simulink library "tp333079"  (Simulink 5.0)
values from neighbouring files (symbols this model uses):
  b = 1    [main_flock3.m]    (also in main_flock4.m; params_flocking_ros.m)
undefined symbols (not defined in the file or in its folder): AC, AlphaBnd, BetaBnd, CDda, CDde, CDdf, CDdr, CDM, CDmin, CGempty, CGgross, CL0, CLa, CLalphadot, Clbeta, Clda, CLde, CLdf, Cldr, CLM, CLmind, Clp, CLq, Clr, Cm0, Cma, Cmalphadot, Cmde, Cmdf, CmM, Cmq, Cnbeta, Cnda, Cndr, Cnp, Cnr, CP, CT, CYbeta, CYda, CYdr, CYp, CYr, Displacement, dmy, Engine, EulerIni, FuelFlow, FuelIni, J, Jempty, Jeng, Jgross, Jprop, MAC, MAP, MAPLim, MassIni, MaxPower, mempty ... (+26)
libraries: aerosimlib x325, simulink3 x42
(part 9 of 11)

== system tp333079/FlightGear-Compatible/Propulsion/Thruster/Propeller ==
  FG Fixed-Pitch Propeller : Subsystem  SimViewingDevice=off  mask(FG Fixed-pitch propeller model){Thr=Thruster}
      mask prompts: Thr "Thruster structure:"
      mask help: Fixed-pitch propeller model using look-up tables of thrust and power coefficients as functions of advance ratio.
      settings: Permissions=ReadWrite  RTWFcnNameOpts=Auto  RTWFileNameOpts=Auto
      mask Help:
      | The block provides a fixed-pitch propeller model based on look-up tables for thrust and power coefficients as function of the advance ratio.
      | <P><B>Inputs:</B>
      | <LI>Airspeed = the current aircraft airspeed</LI>
      | <LI>rho = the air density at current aircraft altitude</LI>
      | <LI>Omega = the propeller rotation speed</LI>
      | </P>
      | <P><B>Output:</B>
      | <LI>Fprop = the thrust force generated by the propeller (on body x-axis)</LI>
      | <LI>Mprop = the moment generated by the propeller (on body x-axis)</LI>
      | <LI>PropCoeff = the 3x1 vector of propeller coefficients [J CT CP]</LI>
      | </P>
      | <P><B>Parameters:</B>
      | <LI>Thruster structure = the thruster structure which is a part of the Matlab structure</LI>
      | </P>
  FG Variable-Pitch Propeller : Subsystem  SimViewingDevice=off  mask(FG Variable-pitch propeller model){Thr=Thr}
      mask prompts: Thr "Thruster structure:"
      mask help: Variable-pitch propeller model using look-up tables of thrust and power coefficients as functions of advance ratio and pitch angle.
      settings: Permissions=ReadWrite  RTWFcnNameOpts=Auto  RTWFileNameOpts=Auto
      mask Help:
      | The block provides a variable-pitch propeller model based on look-up tables for thrust and power coefficients as function of the advance ratio and blade pitch angle.
      | <P><B>Inputs:</B>
      | <LI>Airspeed = the current aircraft airspeed</LI>
      | <LI>rho = the air density at current aircraft altitude</LI>
      | <LI>Omega = the propeller rotation speed</LI>
      | <LI>Pitch = the prop blade pitch angle</LI>
      | </P>
      | <P><B>Output:</B>
      | <LI>Fprop = the thrust force generated by the propeller (on body x-axis)</LI>
      | <LI>Mprop = the moment generated by the propeller (on body x-axis)</LI>
      | <LI>PropCoeff = the 3x1 vector of propeller coefficients [J CT CP]</LI>
      | </P>
      | <P><B>Parameters:</B>
      | <LI>Thruster structure = the thruster structure which is a part of the aircraft structure.</LI>
      | </P>

== system tp333079/Equations of Motion/Body-Frame EOM/Kinematics (Quaternions)/Normalization/Vector norm ==
  Vec : Inport  Port=1  PortDimensions=-1  SampleTime=-1  DataType=auto
      settings: SignalType=auto
  Dot Product : simulink3/Math/Dot Product
  Math Function : Math  Operator=sqrt  OutputSignalType=auto
  Mag : Outport  Port=1
  wires:
  Math Function/1 -> Mag/1
  Dot Product/1 -> Math Function/1
  Vec/1 -> Dot Product/2, Dot Product/1

== system tp333079/FlightGear-Compatible/Complete Aircraft/CESSNA-172/Aerodynamics/Drag ==
  Control : Inport  Port=1  PortDimensions=[4 1]  SampleTime=-1  DataType=auto
      settings: SignalType=auto
  WindAxesVel : Inport  Port=2  PortDimensions=[3 1]  SampleTime=-1  DataType=auto
      settings: SignalType=auto
  GndEffect : Inport  Port=3  PortDimensions=1  SampleTime=-1  DataType=auto
      settings: SignalType=auto
  CD alpha : Subsystem  BlockChoice=Table  SimViewingDevice=off
      link override Table: Table=AC.Aerodynamics.Drag.Basic.CDwbh
      link override Value: Value=AC.Aerodynamics.Lift.Basic.kCLge
      link override Vector: Vector=AC.Aerodynamics.Lift.Basic.CLDf
      settings: AttributesFormatString=%<BlockChoice>  TemplateBlock=aerosimlib/FlightGear-Compatible/Aerodynamics/Coefficient  MemberBlocks=Table,Value,Vector  Permissions=ReadWrite  RTWFcnNameOpts=Auto  RTWFileNameOpts=Auto
  CD beta : Subsystem  BlockChoice=Value  SimViewingDevice=off
      link override Value: Value=AC.Aerodynamics.Drag.CDbeta
      settings: AttributesFormatString=%<BlockChoice>  TemplateBlock=aerosimlib/FlightGear-Compatible/Aerodynamics/Coefficient  MemberBlocks=Table,Value,Vector  Permissions=ReadWrite  RTWFcnNameOpts=Auto  RTWFileNameOpts=Auto
  CD elevator : Subsystem  BlockChoice=Value  SimViewingDevice=off
      link override Value: Value=AC.Aerodynamics.Drag.CDDe
      settings: AttributesFormatString=%<BlockChoice>  TemplateBlock=aerosimlib/FlightGear-Compatible/Aerodynamics/Coefficient  MemberBlocks=Table,Value,Vector  Permissions=ReadWrite  RTWFcnNameOpts=Auto  RTWFileNameOpts=Auto
  CD flap : Subsystem  BlockChoice=Vector  SimViewingDevice=off
      link override Value: Value=AC.Aerodynamics.Lift.Basic.kCLge
      link override Vector: Vector=AC.Aerodynamics.Drag.Basic.CDDf
      settings: AttributesFormatString=%<BlockChoice>  TemplateBlock=aerosimlib/FlightGear-Compatible/Aerodynamics/Coefficient  MemberBlocks=Table,Value,Vector  Permissions=ReadWrite  RTWFcnNameOpts=Auto  RTWFileNameOpts=Auto
  CDo : Constant  Value=AC.Aerodynamics.Drag.CDo.Data
  Demux : Demux  Outputs=4  BusSelectionMode=off
  Demux1 : Demux  Outputs=3  BusSelectionMode=off
  Product : Product  Inputs=2  Multiplication=Element-wise(.*)  SaturateOnIntegerOverflow=on
  Sum : Sum  Inputs=++  SaturateOnIntegerOverflow=on
  Sum1 : Sum  Inputs=++++  SaturateOnIntegerOverflow=on
  Terminator : Terminator
  Terminator1 : Terminator
  Terminator5 : Terminator
  kCD ground effect : Subsystem  BlockChoice=Vector  SimViewingDevice=off
      link override Value: Value=AC.Aerodynamics.Lift.Basic.kCLge
      link override Vector: Vector=AC.Aerodynamics.Drag.Basic.kCDge
      settings: AttributesFormatString=%<BlockChoice>  TemplateBlock=aerosimlib/FlightGear-Compatible/Aerodynamics/Coefficient  MemberBlocks=Table,Value,Vector  Permissions=ReadWrite  RTWFcnNameOpts=Auto  RTWFileNameOpts=Auto
  CD : Outport  Port=1
  wires:
  Demux/2 -> CD elevator/1(RowParam)
  WindAxesVel/1 -> Demux1/1
  Control/1 -> Demux/1
  Demux/1 -> CD alpha/2(ColParam), CD flap/1(RowParam)
  Demux/3 -> Terminator/1
  Demux/4 -> Terminator1/1
  Demux1/3 -> CD alpha/1(RowParam)
  CD alpha/1(Coeff) -> Sum/1
  CD flap/1(Coeff) -> Sum/2
  Sum/1 -> Product/1
  kCD ground effect/1(Coeff) -> Product/2
  Product/1 -> Sum1/1
  CDo/1 -> Sum1/2
  CD elevator/1(Coeff) -> Sum1/3
  CD beta/1(Coeff) -> Sum1/4
  Sum1/1 -> CD/1
  Demux1/1 -> Terminator5/1
  Demux1/2 -> CD beta/1(RowParam)
  GndEffect/1 -> kCD ground effect/1(RowParam)

== system tp333079/FlightGear-Compatible/Complete Aircraft/CESSNA-172/Aerodynamics/Lift ==
  Control : Inport  Port=1  PortDimensions=[4 1]  SampleTime=-1  DataType=auto
      settings: SignalType=auto
  WindAxesVel : Inport  Port=2  PortDimensions=[3 1]  SampleTime=-1  DataType=auto
      settings: SignalType=auto
  AlphaBetaDot : Inport  Port=3  PortDimensions=[2 1]  SampleTime=-1  DataType=auto
      settings: SignalType=auto
  AngularRates : Inport  Port=4  PortDimensions=[3 1]  SampleTime=-1  DataType=auto
      settings: SignalType=auto
  HystParam : Inport  Port=5  PortDimensions=1  SampleTime=-1  DataType=auto
      settings: SignalType=auto
  GndEffect : Inport  Port=6  PortDimensions=1  SampleTime=-1  DataType=auto
      settings: SignalType=auto
  2 : Gain  Gain=2  Multiplication=Element-wise(K.*u)  SaturateOnIntegerOverflow=on
  CL alpha : Subsystem  BlockChoice=Table  SimViewingDevice=off
      link override Table: Table=AC.Aerodynamics.Lift.Basic.CLwbh
      link override Value: Value=AC.Aerodynamics.Lift.Basic.kCLge
      link override Vector: Vector=AC.Aerodynamics.Lift.Basic.CLDf
      settings: AttributesFormatString=%<BlockChoice>  TemplateBlock=aerosimlib/FlightGear-Compatible/Aerodynamics/Coefficient  MemberBlocks=Table,Value,Vector  Permissions=ReadWrite  RTWFcnNameOpts=Auto  RTWFileNameOpts=Auto
  CL elevator : Subsystem  BlockChoice=Value  SimViewingDevice=off
      link override Value: Value=AC.Aerodynamics.Lift.CLDe
      settings: AttributesFormatString=%<BlockChoice>  TemplateBlock=aerosimlib/FlightGear-Compatible/Aerodynamics/Coefficient  MemberBlocks=Table,Value,Vector  Permissions=ReadWrite  RTWFcnNameOpts=Auto  RTWFileNameOpts=Auto
  CL flap : Subsystem  BlockChoice=Vector  SimViewingDevice=off
      link override Value: Value=AC.Aerodynamics.Lift.Basic.kCLge
      link override Vector: Vector=AC.Aerodynamics.Lift.Basic.CLDf
      settings: AttributesFormatString=%<BlockChoice>  TemplateBlock=aerosimlib/FlightGear-Compatible/Aerodynamics/Coefficient  MemberBlocks=Table,Value,Vector  Permissions=ReadWrite  RTWFcnNameOpts=Auto  RTWFileNameOpts=Auto
  CL*c/(2V) : Product  Inputs=**/  Multiplication=Element-wise(.*)  SaturateOnIntegerOverflow=on
  CLalphadot : Subsystem  BlockChoice=Value  SimViewingDevice=off
      link override Value: Value=AC.Aerodynamics.Lift.CLadot
      settings: AttributesFormatString=%<BlockChoice>  TemplateBlock=aerosimlib/FlightGear-Compatible/Aerodynamics/Coefficient  MemberBlocks=Table,Value,Vector  Permissions=ReadWrite  RTWFcnNameOpts=Auto  RTWFileNameOpts=Auto
  CLq : Subsystem  BlockChoice=Value  SimViewingDevice=off
      link override Value: Value=AC.Aerodynamics.Lift.CLq
      settings: AttributesFormatString=%<BlockChoice>  TemplateBlock=aerosimlib/FlightGear-Compatible/Aerodynamics/Coefficient  MemberBlocks=Table,Value,Vector  Permissions=ReadWrite  RTWFcnNameOpts=Auto  RTWFileNameOpts=Auto
  Demux : Demux  Outputs=4  BusSelectionMode=off
  Demux1 : Demux  Outputs=3  BusSelectionMode=off
  Demux2 : Demux  Outputs=2  BusSelectionMode=off
  Demux3 : Demux  Outputs=3  BusSelectionMode=off
  Product : Product  Inputs=2  Multiplication=Element-wise(.*)  SaturateOnIntegerOverflow=on
  Sum : Sum  Inputs=++  SaturateOnIntegerOverflow=on
  Sum1 : Sum  Inputs=+++  SaturateOnIntegerOverflow=on
  Sum2 : Sum  Inputs=++  SaturateOnIntegerOverflow=on
  Terminator{,1..4,6} (6 alike) : Terminator
  Wing chord : Constant  Value=AC.Metrics.WingChord
  kCL ground effect : Subsystem  BlockChoice=Vector  SimViewingDevice=off
      link override Value: Value=AC.Aerodynamics.Lift.Basic.kCLge
      link override Vector: Vector=AC.Aerodynamics.Lift.Basic.kCLge
      settings: AttributesFormatString=%<BlockChoice>  TemplateBlock=aerosimlib/FlightGear-Compatible/Aerodynamics/Coefficient  MemberBlocks=Table,Value,Vector  Permissions=ReadWrite  RTWFcnNameOpts=Auto  RTWFileNameOpts=Auto
  CL : Outport  Port=1
  wires:
  CL*c/(2V)/1 -> Sum1/3
  CLq/1(Coeff) -> Sum2/2
  CLalphadot/1(Coeff) -> Sum2/1
  Sum2/1 -> CL*c/(2V)/1
  Wing chord/1 -> CL*c/(2V)/2
  2/1 -> CL*c/(2V)/3
  GndEffect/1 -> kCL ground effect/1(RowParam)
  HystParam/1 -> CL alpha/2(ColParam)
  Demux1/2 -> Terminator6/1
  Demux1/1 -> 2/1
  Sum1/1 -> CL/1
  CL elevator/1(Coeff) -> Sum1/2
  Product/1 -> Sum1/1
  kCL ground effect/1(Coeff) -> Product/2
  Sum/1 -> Product/1
  CL flap/1(Coeff) -> Sum/2
  CL alpha/1(Coeff) -> Sum/1
  Demux3/3 -> Terminator4/1
  Demux3/1 -> Terminator3/1
  Demux2/2 -> Terminator2/1
  Demux3/2 -> CLq/1(RowParam)
  Demux2/1 -> CLalphadot/1(RowParam)
  Demux1/3 -> CL alpha/1(RowParam)
  Demux/4 -> Terminator1/1
  Demux/3 -> Terminator/1
  Demux/2 -> CL elevator/1(RowParam)
  Demux/1 -> CL flap/1(RowParam)
  AngularRates/1 -> Demux3/1
  AlphaBetaDot/1 -> Demux2/1
  Control/1 -> Demux/1
  WindAxesVel/1 -> Demux1/1

== system tp333079/FlightGear-Compatible/Complete Aircraft/CESSNA-172/Aerodynamics/Pitch ==
  Control : Inport  Port=1  PortDimensions=[4 1]  SampleTime=-1  DataType=auto
      settings: SignalType=auto
  WindAxesVel : Inport  Port=2  PortDimensions=[3 1]  SampleTime=-1  DataType=auto
      settings: SignalType=auto
  AlphaBetaDot : Inport  Port=3  PortDimensions=[2 1]  SampleTime=-1  DataType=auto
      settings: SignalType=auto
  AngularRates : Inport  Port=4  PortDimensions=[3 1]  SampleTime=-1  DataType=auto
      settings: SignalType=auto
  2 : Gain  Gain=2  Multiplication=Element-wise(K.*u)  SaturateOnIntegerOverflow=on
  Cm alpha : Subsystem  BlockChoice=Value  SimViewingDevice=off
      link override Table: Table=AC.Aerodynamics.Lift.Basic.CLwbh
      link override Value: Value=AC.Aerodynamics.Pitch.Cmalpha
      link override Vector: Vector=AC.Aerodynamics.Lift.Basic.CLDf
      settings: AttributesFormatString=%<BlockChoice>  TemplateBlock=aerosimlib/FlightGear-Compatible/Aerodynamics/Coefficient  MemberBlocks=Table,Value,Vector  Permissions=ReadWrite  RTWFcnNameOpts=Auto  RTWFileNameOpts=Auto
  Cm elevator : Subsystem  BlockChoice=Value  SimViewingDevice=off
      link override Value: Value=AC.Aerodynamics.Pitch.Cmde
      settings: AttributesFormatString=%<BlockChoice>  TemplateBlock=aerosimlib/FlightGear-Compatible/Aerodynamics/Coefficient  MemberBlocks=Table,Value,Vector  Permissions=ReadWrite  RTWFcnNameOpts=Auto  RTWFileNameOpts=Auto
  Cm flap : Subsystem  BlockChoice=Vector  SimViewingDevice=off
      link override Value: Value=AC.Aerodynamics.Lift.Basic.kCLge
      link override Vector: Vector=AC.Aerodynamics.Pitch.Cmdf
      settings: AttributesFormatString=%<BlockChoice>  TemplateBlock=aerosimlib/FlightGear-Compatible/Aerodynamics/Coefficient  MemberBlocks=Table,Value,Vector  Permissions=ReadWrite  RTWFcnNameOpts=Auto  RTWFileNameOpts=Auto
  Cm*c/(2V) : Product  Inputs=**/  Multiplication=Element-wise(.*)  SaturateOnIntegerOverflow=on
  Cmalphadot : Subsystem  BlockChoice=Value  SimViewingDevice=off
      link override Value: Value=AC.Aerodynamics.Pitch.Cmadot
      settings: AttributesFormatString=%<BlockChoice>  TemplateBlock=aerosimlib/FlightGear-Compatible/Aerodynamics/Coefficient  MemberBlocks=Table,Value,Vector  Permissions=ReadWrite  RTWFcnNameOpts=Auto  RTWFileNameOpts=Auto
  Cmo : Constant  Value=AC.Aerodynamics.Pitch.Cmo.Data
  Cmq : Subsystem  BlockChoice=Value  SimViewingDevice=off
      link override Value: Value=AC.Aerodynamics.Pitch.Cmq
      settings: AttributesFormatString=%<BlockChoice>  TemplateBlock=aerosimlib/FlightGear-Compatible/Aerodynamics/Coefficient  MemberBlocks=Table,Value,Vector  Permissions=ReadWrite  RTWFcnNameOpts=Auto  RTWFileNameOpts=Auto
  Demux : Demux  Outputs=4  BusSelectionMode=off
  Demux1 : Demux  Outputs=3  BusSelectionMode=off
  Demux2 : Demux  Outputs=2  BusSelectionMode=off
  Demux3 : Demux  Outputs=3  BusSelectionMode=off
  Sum1 : Sum  Inputs=+++++  SaturateOnIntegerOverflow=on
  Sum2 : Sum  Inputs=++  SaturateOnIntegerOverflow=on
  Terminator{,1..4,6} (6 alike) : Terminator
  Wing chord : Constant  Value=AC.Metrics.WingChord
  Cm : Outport  Port=1
  wires:
  Cm*c/(2V)/1 -> Sum1/5
  Cm elevator/1(Coeff) -> Sum1/4
  Cmo/1 -> Sum1/3
  Cm flap/1(Coeff) -> Sum1/2
  Cm alpha/1(Coeff) -> Sum1/1
  Demux3/2 -> Cmq/1(RowParam)
  Demux2/1 -> Cmalphadot/1(RowParam)
  Demux1/3 -> Cm alpha/1(RowParam)
  Demux1/1 -> 2/1
  Demux/2 -> Cm elevator/1(RowParam)
  Demux/1 -> Cm flap/1(RowParam)
  WindAxesVel/1 -> Demux1/1
  Control/1 -> Demux/1
  AlphaBetaDot/1 -> Demux2/1
  AngularRates/1 -> Demux3/1
  Demux/3 -> Terminator/1
  Demux/4 -> Terminator1/1
  Demux2/2 -> Terminator2/1
  Demux3/1 -> Terminator3/1
  Demux3/3 -> Terminator4/1
  Sum1/1 -> Cm/1
  Demux1/2 -> Terminator6/1
  2/1 -> Cm*c/(2V)/3
  Wing chord/1 -> Cm*c/(2V)/2
  Sum2/1 -> Cm*c/(2V)/1
  Cmalphadot/1(Coeff) -> Sum2/1
  Cmq/1(Coeff) -> Sum2/2

== system tp333079/FlightGear-Compatible/Complete Aircraft/CESSNA-172/Aerodynamics/Roll ==
  Control : Inport  Port=1  PortDimensions=[4 1]  SampleTime=-1  DataType=auto
      settings: SignalType=auto
  WindAxesVel : Inport  Port=2  PortDimensions=[3 1]  SampleTime=-1  DataType=auto
      settings: SignalType=auto
  AngularRates : Inport  Port=3  PortDimensions=[3 1]  SampleTime=-1  DataType=auto
      settings: SignalType=auto
  2 : Gain  Gain=2  Multiplication=Element-wise(K.*u)  SaturateOnIntegerOverflow=on
  Cl aileron : Subsystem  BlockChoice=Value  SimViewingDevice=off
      link override Value: Value=AC.Aerodynamics.Roll.ClDa
      settings: AttributesFormatString=%<BlockChoice>  TemplateBlock=aerosimlib/FlightGear-Compatible/Aerodynamics/Coefficient  MemberBlocks=Table,Value,Vector  Permissions=ReadWrite  RTWFcnNameOpts=Auto  RTWFileNameOpts=Auto
  Cl beta : Subsystem  BlockChoice=Vector  SimViewingDevice=off
      link override Value: Value=AC.Aerodynamics.Lift.Basic.kCLge
      link override Vector: Vector=AC.Aerodynamics.Roll.Clb
      settings: AttributesFormatString=%<BlockChoice>  TemplateBlock=aerosimlib/FlightGear-Compatible/Aerodynamics/Coefficient  MemberBlocks=Table,Value,Vector  Permissions=ReadWrite  RTWFcnNameOpts=Auto  RTWFileNameOpts=Auto
  Cl rudder : Subsystem  BlockChoice=Value  SimViewingDevice=off
      link override Value: Value=AC.Aerodynamics.Roll.Cldr
      settings: AttributesFormatString=%<BlockChoice>  TemplateBlock=aerosimlib/FlightGear-Compatible/Aerodynamics/Coefficient  MemberBlocks=Table,Value,Vector  Permissions=ReadWrite  RTWFcnNameOpts=Auto  RTWFileNameOpts=Auto
  Cl*b/(2V) : Product  Inputs=**/  Multiplication=Element-wise(.*)  SaturateOnIntegerOverflow=on
  Clp : Subsystem  BlockChoice=Value  SimViewingDevice=off
      link override Value: Value=AC.Aerodynamics.Roll.Clp
      settings: AttributesFormatString=%<BlockChoice>  TemplateBlock=aerosimlib/FlightGear-Compatible/Aerodynamics/Coefficient  MemberBlocks=Table,Value,Vector  Permissions=ReadWrite  RTWFcnNameOpts=Auto  RTWFileNameOpts=Auto
  Clr : Subsystem  BlockChoice=Table  SimViewingDevice=off
      link override Table: Table=AC.Aerodynamics.Roll.Clr
      link override Value: Value=AC.Aerodynamics.Side.CYdr
      link override Vector: Vector=AC.Aerodynamics.Roll.Clr
      settings: AttributesFormatString=%<BlockChoice>  TemplateBlock=aerosimlib/FlightGear-Compatible/Aerodynamics/Coefficient  MemberBlocks=Table,Value,Vector  Permissions=ReadWrite  RTWFcnNameOpts=Auto  RTWFileNameOpts=Auto
  Clr*r : Product  Inputs=2  Multiplication=Element-wise(.*)  SaturateOnIntegerOverflow=on
  Demux : Demux  Outputs=4  BusSelectionMode=off
  Demux1 : Demux  Outputs=3  BusSelectionMode=off
  Demux3 : Demux  Outputs=3  BusSelectionMode=off
  Sum : Sum  Inputs=++  SaturateOnIntegerOverflow=on
  Sum1 : Sum  Inputs=++++  SaturateOnIntegerOverflow=on
  Terminator3 : Terminator
  Terminator4 : Terminator
  Wing span : Constant  Value=AC.Metrics.WingSpan
  Cl : Outport  Port=1
  wires:
  Sum1/1 -> Cl/1
  AngularRates/1 -> Demux3/1
  Control/1 -> Demux/1
  WindAxesVel/1 -> Demux1/1
  Clp/1(Coeff) -> Sum/1
  Wing span/1 -> Cl*b/(2V)/2
  2/1 -> Cl*b/(2V)/3
  Sum/1 -> Cl*b/(2V)/1
  Demux1/1 -> 2/1
  Demux1/2 -> Cl beta/1(RowParam)
  Demux/3 -> Cl aileron/1(RowParam)
  Demux/4 -> Cl rudder/1(RowParam)
  Demux3/1 -> Clp/1(RowParam)
  Demux3/2 -> Terminator4/1
  Demux1/3 -> Clr/1(RowParam)
  Demux/1 -> Clr/2(ColParam)
  Demux/2 -> Terminator3/1
  Cl beta/1(Coeff) -> Sum1/1
  Cl aileron/1(Coeff) -> Sum1/2
  Cl rudder/1(Coeff) -> Sum1/3
  Cl*b/(2V)/1 -> Sum1/4
  Clr*r/1 -> Sum/2
  Clr/1(Coeff) -> Clr*r/1
  Demux3/3 -> Clr*r/2

== system tp333079/FlightGear-Compatible/Complete Aircraft/CESSNA-172/Aerodynamics/Side ==
  Control : Inport  Port=1  PortDimensions=[4 1]  SampleTime=-1  DataType=auto
      settings: SignalType=auto
  WindAxesVel : Inport  Port=2  PortDimensions=[3 1]  SampleTime=-1  DataType=auto
      settings: SignalType=auto
  AngularRates : Inport  Port=3  PortDimensions=[3 1]  SampleTime=-1  DataType=auto
      settings: SignalType=auto
  2 : Gain  Gain=2  Multiplication=Element-wise(K.*u)  SaturateOnIntegerOverflow=on
  CY aileron : Subsystem  BlockChoice=Value  SimViewingDevice=off
      link override Value: Value=AC.Aerodynamics.Side.CYda
      settings: AttributesFormatString=%<BlockChoice>  TemplateBlock=aerosimlib/FlightGear-Compatible/Aerodynamics/Coefficient  MemberBlocks=Table,Value,Vector  Permissions=ReadWrite  RTWFcnNameOpts=Auto  RTWFileNameOpts=Auto
  CY beta : Subsystem  BlockChoice=Table  SimViewingDevice=off
      link override Table: Table=AC.Aerodynamics.Side.CYb
      link override Value: Value=AC.Aerodynamics.Lift.Basic.kCLge
      link override Vector: Vector=AC.Aerodynamics.Side.CYb
      settings: AttributesFormatString=%<BlockChoice>  TemplateBlock=aerosimlib/FlightGear-Compatible/Aerodynamics/Coefficient  MemberBlocks=Table,Value,Vector  Permissions=ReadWrite  RTWFcnNameOpts=Auto  RTWFileNameOpts=Auto
  CY rudder : Subsystem  BlockChoice=Value  SimViewingDevice=off
      link override Value: Value=AC.Aerodynamics.Side.CYdr
      settings: AttributesFormatString=%<BlockChoice>  TemplateBlock=aerosimlib/FlightGear-Compatible/Aerodynamics/Coefficient  MemberBlocks=Table,Value,Vector  Permissions=ReadWrite  RTWFcnNameOpts=Auto  RTWFileNameOpts=Auto
  CY*b/(2V) : Product  Inputs=**/  Multiplication=Element-wise(.*)  SaturateOnIntegerOverflow=on
  CYp : Subsystem  BlockChoice=Table  SimViewingDevice=off
      link override Table: Table=AC.Aerodynamics.Side.CYp
      link override Value: Value=AC.Aerodynamics.Side.CYp
      settings: AttributesFormatString=%<BlockChoice>  TemplateBlock=aerosimlib/FlightGear-Compatible/Aerodynamics/Coefficient  MemberBlocks=Table,Value,Vector  Permissions=ReadWrite  RTWFcnNameOpts=Auto  RTWFileNameOpts=Auto
  CYr : Subsystem  BlockChoice=Table  SimViewingDevice=off
      link override Table: Table=AC.Aerodynamics.Side.CYr
      link override Value: Value=AC.Aerodynamics.Side.CYr
      settings: AttributesFormatString=%<BlockChoice>  TemplateBlock=aerosimlib/FlightGear-Compatible/Aerodynamics/Coefficient  MemberBlocks=Table,Value,Vector  Permissions=ReadWrite  RTWFcnNameOpts=Auto  RTWFileNameOpts=Auto
  Demux : Demux  Outputs=4  BusSelectionMode=off
  Demux1 : Demux  Outputs=3  BusSelectionMode=off
  Demux3 : Demux  Outputs=3  BusSelectionMode=off
  Product : Product  Inputs=2  Multiplication=Element-wise(.*)  SaturateOnIntegerOverflow=on
  Product1 : Product  Inputs=2  Multiplication=Element-wise(.*)  SaturateOnIntegerOverflow=on
  Sum : Sum  Inputs=++  SaturateOnIntegerOverflow=on
  Sum1 : Sum  Inputs=++++  SaturateOnIntegerOverflow=on
  Terminator3 : Terminator
  Terminator4 : Terminator
  Wing span : Constant  Value=AC.Metrics.WingSpan
  CY : Outport  Port=1
  wires:
  CY*b/(2V)/1 -> Sum1/4
  CY rudder/1(Coeff) -> Sum1/3
  CY aileron/1(Coeff) -> Sum1/2
  CY beta/1(Coeff) -> Sum1/1
  Demux/2 -> Terminator3/1
  Demux/1 -> CY beta/2(ColParam), CYp/2(ColParam), CYr/2(ColParam)
  Demux1/3 -> CYp/1(RowParam), CYr/1(RowParam)
  Demux3/2 -> Terminator4/1
  Demux/4 -> CY rudder/1(RowParam)
  Demux/3 -> CY aileron/1(RowParam)
  Demux1/2 -> CY beta/1(RowParam)
  Demux1/1 -> 2/1
  Sum/1 -> CY*b/(2V)/1
  2/1 -> CY*b/(2V)/3
  Wing span/1 -> CY*b/(2V)/2
  WindAxesVel/1 -> Demux1/1
  Control/1 -> Demux/1
  AngularRates/1 -> Demux3/1
  Sum1/1 -> CY/1
  Product/1 -> Sum/1
  Product1/1 -> Sum/2
  CYp/1(Coeff) -> Product/1
  CYr/1(Coeff) -> Product1/1
  Demux3/1 -> Product/2
  Demux3/3 -> Product1/2

== system tp333079/FlightGear-Compatible/Complete Aircraft/CESSNA-172/Aerodynamics/Yaw ==
  Control : Inport  Port=1  PortDimensions=[4 1]  SampleTime=-1  DataType=auto
      settings: SignalType=auto
  WindAxesVel : Inport  Port=2  PortDimensions=[3 1]  SampleTime=-1  DataType=auto
      settings: SignalType=auto
  AngularRates : Inport  Port=3  PortDimensions=[3 1]  SampleTime=-1  DataType=auto
      settings: SignalType=auto
  2 : Gain  Gain=2  Multiplication=Element-wise(K.*u)  SaturateOnIntegerOverflow=on
  Cn aileron : Subsystem  BlockChoice=Value  SimViewingDevice=off
      link override Value: Value=AC.Aerodynamics.Yaw.Cnda
      settings: AttributesFormatString=%<BlockChoice>  TemplateBlock=aerosimlib/FlightGear-Compatible/Aerodynamics/Coefficient  MemberBlocks=Table,Value,Vector  Permissions=ReadWrite  RTWFcnNameOpts=Auto  RTWFileNameOpts=Auto
  Cn beta : Subsystem  BlockChoice=Vector  SimViewingDevice=off
      link override Value: Value=AC.Aerodynamics.Lift.Basic.kCLge
      link override Vector: Vector=AC.Aerodynamics.Yaw.Cnb
      settings: AttributesFormatString=%<BlockChoice>  TemplateBlock=aerosimlib/FlightGear-Compatible/Aerodynamics/Coefficient  MemberBlocks=Table,Value,Vector  Permissions=ReadWrite  RTWFcnNameOpts=Auto  RTWFileNameOpts=Auto
  Cn rudder : Subsystem  BlockChoice=Value  SimViewingDevice=off
      link override Value: Value=AC.Aerodynamics.Yaw.Cndr
      settings: AttributesFormatString=%<BlockChoice>  TemplateBlock=aerosimlib/FlightGear-Compatible/Aerodynamics/Coefficient  MemberBlocks=Table,Value,Vector  Permissions=ReadWrite  RTWFcnNameOpts=Auto  RTWFileNameOpts=Auto
  Cn*b/(2V) : Product  Inputs=**/  Multiplication=Element-wise(.*)  SaturateOnIntegerOverflow=on
  Cnp : Subsystem  BlockChoice=Value  SimViewingDevice=off
      link override Value: Value=AC.Aerodynamics.Yaw.Cnp
      settings: AttributesFormatString=%<BlockChoice>  TemplateBlock=aerosimlib/FlightGear-Compatible/Aerodynamics/Coefficient  MemberBlocks=Table,Value,Vector  Permissions=ReadWrite  RTWFcnNameOpts=Auto  RTWFileNameOpts=Auto
  Cnr : Subsystem  BlockChoice=Value  SimViewingDevice=off
      link override Value: Value=AC.Aerodynamics.Yaw.Cnr
      link override Vector: Vector=AC.Aerodynamics.Roll.Clr
      settings: AttributesFormatString=%<BlockChoice>  TemplateBlock=aerosimlib/FlightGear-Compatible/Aerodynamics/Coefficient  MemberBlocks=Table,Value,Vector  Permissions=ReadWrite  RTWFcnNameOpts=Auto  RTWFileNameOpts=Auto
  Demux : Demux  Outputs=4  BusSelectionMode=off
  Demux1 : Demux  Outputs=3  BusSelectionMode=off
  Demux3 : Demux  Outputs=3  BusSelectionMode=off
  Sum : Sum  Inputs=++  SaturateOnIntegerOverflow=on
  Sum1 : Sum  Inputs=++++  SaturateOnIntegerOverflow=on
  Terminator{1..4} (4 alike) : Terminator
  Wing span : Constant  Value=AC.Metrics.WingSpan
  Cn : Outport  Port=1
  wires:
  Cn*b/(2V)/1 -> Sum1/4
  Cn rudder/1(Coeff) -> Sum1/3
  Cn aileron/1(Coeff) -> Sum1/2
  Cn beta/1(Coeff) -> Sum1/1
  Demux/2 -> Terminator3/1
  Demux/1 -> Terminator2/1
  Demux1/3 -> Terminator1/1
  Demux3/2 -> Terminator4/1
  Demux3/3 -> Cnr/1(RowParam)
  Demux3/1 -> Cnp/1(RowParam)
  Demux/4 -> Cn rudder/1(RowParam)
  Demux/3 -> Cn aileron/1(RowParam)
  Demux1/2 -> Cn beta/1(RowParam)
  Demux1/1 -> 2/1
  Sum/1 -> Cn*b/(2V)/1
  2/1 -> Cn*b/(2V)/3
  Wing span/1 -> Cn*b/(2V)/2
  Cnr/1(Coeff) -> Sum/2
  Cnp/1(Coeff) -> Sum/1
  WindAxesVel/1 -> Demux1/1
  Control/1 -> Demux/1
  AngularRates/1 -> Demux3/1
  Sum1/1 -> Cn/1

== system tp333079/FlightGear-Compatible/Complete Aircraft/CESSNA-182/Aerodynamics/Drag ==
  Control : Inport  Port=1  PortDimensions=[4 1]  SampleTime=-1  DataType=auto
      settings: SignalType=auto
  WindAxesVel : Inport  Port=2  PortDimensions=[3 1]  SampleTime=-1  DataType=auto
      settings: SignalType=auto
  CD alpha : Subsystem  BlockChoice=Vector  SimViewingDevice=off
      link override Table: Table=AC.Aerodynamics.Drag.Basic.CDwbh
      link override Value: Value=AC.Aerodynamics.Lift.Basic.kCLge
      link override Vector: Vector=AC.Aerodynamics.Drag.CDalpha
      settings: AttributesFormatString=%<BlockChoice>  TemplateBlock=aerosimlib/FlightGear-Compatible/Aerodynamics/Coefficient  MemberBlocks=Table,Value,Vector  Permissions=ReadWrite  RTWFcnNameOpts=Auto  RTWFileNameOpts=Auto
  CD beta : Subsystem  BlockChoice=Value  SimViewingDevice=off
      link override Value: Value=AC.Aerodynamics.Drag.CDbeta
      settings: AttributesFormatString=%<BlockChoice>  TemplateBlock=aerosimlib/FlightGear-Compatible/Aerodynamics/Coefficient  MemberBlocks=Table,Value,Vector  Permissions=ReadWrite  RTWFcnNameOpts=Auto  RTWFileNameOpts=Auto
  CD elevator : Subsystem  BlockChoice=Value  SimViewingDevice=off
      link override Value: Value=AC.Aerodynamics.Drag.CDDe
      settings: AttributesFormatString=%<BlockChoice>  TemplateBlock=aerosimlib/FlightGear-Compatible/Aerodynamics/Coefficient  MemberBlocks=Table,Value,Vector  Permissions=ReadWrite  RTWFcnNameOpts=Auto  RTWFileNameOpts=Auto
  CD flap : Subsystem  BlockChoice=Table  SimViewingDevice=off
      link override Table: Table=AC.Aerodynamics.Drag.CDDf
      link override Value: Value=AC.Aerodynamics.Lift.Basic.kCLge
      link override Vector: Vector=AC.Aerodynamics.Drag.Basic.CDDf
      settings: AttributesFormatString=%<BlockChoice>  TemplateBlock=aerosimlib/FlightGear-Compatible/Aerodynamics/Coefficient  MemberBlocks=Table,Value,Vector  Permissions=ReadWrite  RTWFcnNameOpts=Auto  RTWFileNameOpts=Auto
  CDo : Constant  Value=AC.Aerodynamics.Drag.CDo.Data
  Demux : Demux  Outputs=4  BusSelectionMode=off
  Demux1 : Demux  Outputs=3  BusSelectionMode=off
  Sum : Sum  Inputs=++  SaturateOnIntegerOverflow=on
  Sum1 : Sum  Inputs=++++  SaturateOnIntegerOverflow=on
  Terminator : Terminator
  Terminator1 : Terminator
  Terminator5 : Terminator
  CD : Outport  Port=1
  wires:
  Demux/1 -> CD flap/2(ColParam)
  Demux/2 -> CD elevator/1(RowParam)
  WindAxesVel/1 -> Demux1/1
  Control/1 -> Demux/1
  Demux/3 -> Terminator/1
  Demux/4 -> Terminator1/1
  Demux1/3 -> CD flap/1(RowParam), CD alpha/1(RowParam)
  CD alpha/1(Coeff) -> Sum/1
  CD flap/1(Coeff) -> Sum/2
  Sum/1 -> Sum1/1
  CDo/1 -> Sum1/2
  CD elevator/1(Coeff) -> Sum1/3
  CD beta/1(Coeff) -> Sum1/4
  Sum1/1 -> CD/1
  Demux1/1 -> Terminator5/1
  Demux1/2 -> CD beta/1(RowParam)

== system tp333079/FlightGear-Compatible/Complete Aircraft/CESSNA-182/Aerodynamics/Lift ==
  Control : Inport  Port=1  PortDimensions=[4 1]  SampleTime=-1  DataType=auto
      settings: SignalType=auto
  WindAxesVel : Inport  Port=2  PortDimensions=[3 1]  SampleTime=-1  DataType=auto
      settings: SignalType=auto
  AlphaBetaDot : Inport  Port=3  PortDimensions=[2 1]  SampleTime=-1  DataType=auto
      settings: SignalType=auto
  AngularRates : Inport  Port=4  PortDimensions=[3 1]  SampleTime=-1  DataType=auto
      settings: SignalType=auto
  GndEffect : Inport  Port=5  PortDimensions=1  SampleTime=-1  DataType=auto
      settings: SignalType=auto
  2 : Gain  Gain=2  Multiplication=Element-wise(K.*u)  SaturateOnIntegerOverflow=on
  CL alpha : Subsystem  BlockChoice=Vector  SimViewingDevice=off
      link override Table: Table=AC.Aerodynamics.Lift.Basic.CLalpha
      link override Value: Value=AC.Aerodynamics.Lift.Basic.kCLge
      link override Vector: Vector=AC.Aerodynamics.Lift.Basic.CLalpha
      settings: AttributesFormatString=%<BlockChoice>  TemplateBlock=aerosimlib/FlightGear-Compatible/Aerodynamics/Coefficient  MemberBlocks=Table,Value,Vector  Permissions=ReadWrite  RTWFcnNameOpts=Auto  RTWFileNameOpts=Auto
  CL elevator : Subsystem  BlockChoice=Value  SimViewingDevice=off
      link override Value: Value=AC.Aerodynamics.Lift.CLDe
      settings: AttributesFormatString=%<BlockChoice>  TemplateBlock=aerosimlib/FlightGear-Compatible/Aerodynamics/Coefficient  MemberBlocks=Table,Value,Vector  Permissions=ReadWrite  RTWFcnNameOpts=Auto  RTWFileNameOpts=Auto
  CL flap : Subsystem  BlockChoice=Vector  SimViewingDevice=off
      link override Value: Value=AC.Aerodynamics.Lift.Basic.kCLge
      link override Vector: Vector=AC.Aerodynamics.Lift.Basic.CLDf
      settings: AttributesFormatString=%<BlockChoice>  TemplateBlock=aerosimlib/FlightGear-Compatible/Aerodynamics/Coefficient  MemberBlocks=Table,Value,Vector  Permissions=ReadWrite  RTWFcnNameOpts=Auto  RTWFileNameOpts=Auto
  CL*c/(2V) : Product  Inputs=**/  Multiplication=Element-wise(.*)  SaturateOnIntegerOverflow=on
  CLalphadot : Subsystem  BlockChoice=Value  SimViewingDevice=off
      link override Value: Value=AC.Aerodynamics.Lift.CLadot
      settings: AttributesFormatString=%<BlockChoice>  TemplateBlock=aerosimlib/FlightGear-Compatible/Aerodynamics/Coefficient  MemberBlocks=Table,Value,Vector  Permissions=ReadWrite  RTWFcnNameOpts=Auto  RTWFileNameOpts=Auto
  CLo : Constant  Value=AC.Aerodynamics.Lift.Basic.CLo.Data
  CLq : Subsystem  BlockChoice=Value  SimViewingDevice=off
      link override Value: Value=AC.Aerodynamics.Lift.CLq
      settings: AttributesFormatString=%<BlockChoice>  TemplateBlock=aerosimlib/FlightGear-Compatible/Aerodynamics/Coefficient  MemberBlocks=Table,Value,Vector  Permissions=ReadWrite  RTWFcnNameOpts=Auto  RTWFileNameOpts=Auto
  Demux : Demux  Outputs=4  BusSelectionMode=off
  Demux1 : Demux  Outputs=3  BusSelectionMode=off
  Demux2 : Demux  Outputs=2  BusSelectionMode=off
  Demux3 : Demux  Outputs=3  BusSelectionMode=off
  Product : Product  Inputs=2  Multiplication=Element-wise(.*)  SaturateOnIntegerOverflow=on
  Sum : Sum  Inputs=+++  SaturateOnIntegerOverflow=on
  Sum1 : Sum  Inputs=+++  SaturateOnIntegerOverflow=on
  Sum2 : Sum  Inputs=++  SaturateOnIntegerOverflow=on
  Terminator{,1..4,6} (6 alike) : Terminator
  Wing chord : Constant  Value=AC.Metrics.WingChord
  kCL ground effect : Subsystem  BlockChoice=Vector  SimViewingDevice=off
      link override Value: Value=AC.Aerodynamics.Lift.Basic.kCLge
      link override Vector: Vector=AC.Aerodynamics.Lift.Basic.kCLge
      settings: AttributesFormatString=%<BlockChoice>  TemplateBlock=aerosimlib/FlightGear-Compatible/Aerodynamics/Coefficient  MemberBlocks=Table,Value,Vector  Permissions=ReadWrite  RTWFcnNameOpts=Auto  RTWFileNameOpts=Auto
  CL : Outport  Port=1
  wires:
  CLo/1 -> Sum/3
  CL*c/(2V)/1 -> Sum1/3
  CLq/1(Coeff) -> Sum2/2
  CLalphadot/1(Coeff) -> Sum2/1
  Sum2/1 -> CL*c/(2V)/1
  Wing chord/1 -> CL*c/(2V)/2
  2/1 -> CL*c/(2V)/3
  GndEffect/1 -> kCL ground effect/1(RowParam)
  Demux1/2 -> Terminator6/1
  Demux1/1 -> 2/1
  Sum1/1 -> CL/1
  CL elevator/1(Coeff) -> Sum1/2
  Product/1 -> Sum1/1
  kCL ground effect/1(Coeff) -> Product/2
  Sum/1 -> Product/1
  CL flap/1(Coeff) -> Sum/2
  CL alpha/1(Coeff) -> Sum/1
  Demux3/3 -> Terminator4/1
  Demux3/1 -> Terminator3/1
  Demux2/2 -> Terminator2/1
  Demux3/2 -> CLq/1(RowParam)
  Demux2/1 -> CLalphadot/1(RowParam)
  Demux1/3 -> CL alpha/1(RowParam)
  Demux/4 -> Terminator1/1
  Demux/3 -> Terminator/1
  Demux/2 -> CL elevator/1(RowParam)
  Demux/1 -> CL flap/1(RowParam)
  AngularRates/1 -> Demux3/1
  AlphaBetaDot/1 -> Demux2/1
  Control/1 -> Demux/1
  WindAxesVel/1 -> Demux1/1

== system tp333079/FlightGear-Compatible/Complete Aircraft/CESSNA-182/Aerodynamics/Pitch ==
  Control : Inport  Port=1  PortDimensions=[4 1]  SampleTime=-1  DataType=auto
      settings: SignalType=auto
  WindAxesVel : Inport  Port=2  PortDimensions=[3 1]  SampleTime=-1  DataType=auto
      settings: SignalType=auto
  AlphaBetaDot : Inport  Port=3  PortDimensions=[2 1]  SampleTime=-1  DataType=auto
      settings: SignalType=auto
  AngularRates : Inport  Port=4  PortDimensions=[3 1]  SampleTime=-1  DataType=auto
      settings: SignalType=auto
  2 : Gain  Gain=2  Multiplication=Element-wise(K.*u)  SaturateOnIntegerOverflow=on
  Cm alpha : Subsystem  BlockChoice=Vector  SimViewingDevice=off
      link override Table: Table=AC.Aerodynamics.Lift.Basic.CLwbh
      link override Value: Value=AC.Aerodynamics.Pitch.Cmalpha
      link override Vector: Vector=AC.Aerodynamics.Pitch.Cmalpha
      settings: AttributesFormatString=%<BlockChoice>  TemplateBlock=aerosimlib/FlightGear-Compatible/Aerodynamics/Coefficient  MemberBlocks=Table,Value,Vector  Permissions=ReadWrite  RTWFcnNameOpts=Auto  RTWFileNameOpts=Auto
  Cm elevator : Subsystem  BlockChoice=Vector  SimViewingDevice=off
      link override Value: Value=AC.Aerodynamics.Pitch.CmDe
      link override Vector: Vector=AC.Aerodynamics.Pitch.CmDe
      settings: AttributesFormatString=%<BlockChoice>  TemplateBlock=aerosimlib/FlightGear-Compatible/Aerodynamics/Coefficient  MemberBlocks=Table,Value,Vector  Permissions=ReadWrite  RTWFcnNameOpts=Auto  RTWFileNameOpts=Auto
  Cm flap : Subsystem  BlockChoice=Vector  SimViewingDevice=off
      link override Value: Value=AC.Aerodynamics.Lift.Basic.kCLge
      link override Vector: Vector=AC.Aerodynamics.Pitch.CmDf
      settings: AttributesFormatString=%<BlockChoice>  TemplateBlock=aerosimlib/FlightGear-Compatible/Aerodynamics/Coefficient  MemberBlocks=Table,Value,Vector  Permissions=ReadWrite  RTWFcnNameOpts=Auto  RTWFileNameOpts=Auto
  Cm*c/(2V) : Product  Inputs=**/  Multiplication=Element-wise(.*)  SaturateOnIntegerOverflow=on
  Cma*a : Product  Inputs=2  Multiplication=Element-wise(.*)  SaturateOnIntegerOverflow=on
  Cma*a1 : Product  Inputs=2  Multiplication=Element-wise(.*)  SaturateOnIntegerOverflow=on
  Cma*a2 : Product  Inputs=2  Multiplication=Element-wise(.*)  SaturateOnIntegerOverflow=on
  Cmalphadot : Subsystem  BlockChoice=Vector  SimViewingDevice=off
      link override Value: Value=AC.Aerodynamics.Pitch.Cmadot
      link override Vector: Vector=AC.Aerodynamics.Pitch.Cmadot
      settings: AttributesFormatString=%<BlockChoice>  TemplateBlock=aerosimlib/FlightGear-Compatible/Aerodynamics/Coefficient  MemberBlocks=Table,Value,Vector  Permissions=ReadWrite  RTWFcnNameOpts=Auto  RTWFileNameOpts=Auto
  Cmo : Constant  Value=AC.Aerodynamics.Pitch.Cmo.Data
  Cmq : Subsystem  BlockChoice=Value  SimViewingDevice=off
      link override Value: Value=AC.Aerodynamics.Pitch.Cmq
      settings: AttributesFormatString=%<BlockChoice>  TemplateBlock=aerosimlib/FlightGear-Compatible/Aerodynamics/Coefficient  MemberBlocks=Table,Value,Vector  Permissions=ReadWrite  RTWFcnNameOpts=Auto  RTWFileNameOpts=Auto
  Demux : Demux  Outputs=4  BusSelectionMode=off
  Demux1 : Demux  Outputs=3  BusSelectionMode=off
  Demux2 : Demux  Outputs=2  BusSelectionMode=off
  Demux3 : Demux  Outputs=3  BusSelectionMode=off
  Sum1 : Sum  Inputs=+++++  SaturateOnIntegerOverflow=on
  Sum2 : Sum  Inputs=++  SaturateOnIntegerOverflow=on
  Terminator{,1..4,6} (6 alike) : Terminator
  Wing chord : Constant  Value=AC.Metrics.WingChord
  Cm : Outport  Port=1
  wires:
  Cma*a2/1 -> Sum1/4
  Cm elevator/1(Coeff) -> Cma*a2/2
  Demux/2 -> Cma*a2/1
  Demux2/1 -> Cma*a1/2
  Cmalphadot/1(Coeff) -> Cma*a1/1
  Cma*a1/1 -> Sum2/1
  Cm alpha/1(Coeff) -> Cma*a/1
  Cma*a/1 -> Sum1/1
  Cm*c/(2V)/1 -> Sum1/5
  Cmo/1 -> Sum1/3
  Cm flap/1(Coeff) -> Sum1/2
  Demux3/2 -> Cmq/1(RowParam)
  Demux1/3 -> Cm elevator/1(RowParam), Cmalphadot/1(RowParam), Cma*a/2, Cm alpha/1(RowParam)
  Demux1/1 -> 2/1
  Demux/1 -> Cm flap/1(RowParam)
  WindAxesVel/1 -> Demux1/1
  Control/1 -> Demux/1
  AlphaBetaDot/1 -> Demux2/1
  AngularRates/1 -> Demux3/1
  Demux/3 -> Terminator/1
  Demux/4 -> Terminator1/1
  Demux2/2 -> Terminator2/1
  Demux3/1 -> Terminator3/1
  Demux3/3 -> Terminator4/1
  Sum1/1 -> Cm/1
  Demux1/2 -> Terminator6/1
  2/1 -> Cm*c/(2V)/3
  Wing chord/1 -> Cm*c/(2V)/2
  Sum2/1 -> Cm*c/(2V)/1
  Cmq/1(Coeff) -> Sum2/2

== system tp333079/FlightGear-Compatible/Complete Aircraft/CESSNA-182/Aerodynamics/Roll ==
  Control : Inport  Port=1  PortDimensions=[4 1]  SampleTime=-1  DataType=auto
      settings: SignalType=auto
  WindAxesVel : Inport  Port=2  PortDimensions=[3 1]  SampleTime=-1  DataType=auto
      settings: SignalType=auto
  AngularRates : Inport  Port=3  PortDimensions=[3 1]  SampleTime=-1  DataType=auto
      settings: SignalType=auto
  2 : Gain  Gain=2  Multiplication=Element-wise(K.*u)  SaturateOnIntegerOverflow=on
  Cl aileron : Subsystem  BlockChoice=Value  SimViewingDevice=off
      link override Value: Value=AC.Aerodynamics.Roll.ClDa
      settings: AttributesFormatString=%<BlockChoice>  TemplateBlock=aerosimlib/FlightGear-Compatible/Aerodynamics/Coefficient  MemberBlocks=Table,Value,Vector  Permissions=ReadWrite  RTWFcnNameOpts=Auto  RTWFileNameOpts=Auto
  Cl beta : Subsystem  BlockChoice=Table  SimViewingDevice=off
      link override Table: Table=AC.Aerodynamics.Roll.Clb
      link override Value: Value=AC.Aerodynamics.Lift.Basic.kCLge
      link override Vector: Vector=AC.Aerodynamics.Roll.Clb
      settings: AttributesFormatString=%<BlockChoice>  TemplateBlock=aerosimlib/FlightGear-Compatible/Aerodynamics/Coefficient  MemberBlocks=Table,Value,Vector  Permissions=ReadWrite  RTWFcnNameOpts=Auto  RTWFileNameOpts=Auto
  Cl rudder : Subsystem  BlockChoice=Value  SimViewingDevice=off
      link override Value: Value=AC.Aerodynamics.Roll.ClDr
      settings: AttributesFormatString=%<BlockChoice>  TemplateBlock=aerosimlib/FlightGear-Compatible/Aerodynamics/Coefficient  MemberBlocks=Table,Value,Vector  Permissions=ReadWrite  RTWFcnNameOpts=Auto  RTWFileNameOpts=Auto
  Cl*b/(2V) : Product  Inputs=**/  Multiplication=Element-wise(.*)  SaturateOnIntegerOverflow=on
  Clp : Subsystem  BlockChoice=Vector  SimViewingDevice=off
      link override Value: Value=AC.Aerodynamics.Roll.Clp
      link override Vector: Vector=AC.Aerodynamics.Roll.Clp
      settings: AttributesFormatString=%<BlockChoice>  TemplateBlock=aerosimlib/FlightGear-Compatible/Aerodynamics/Coefficient  MemberBlocks=Table,Value,Vector  Permissions=ReadWrite  RTWFcnNameOpts=Auto  RTWFileNameOpts=Auto
  Clp*p : Product  Inputs=2  Multiplication=Element-wise(.*)  SaturateOnIntegerOverflow=on
  Clr : Subsystem  BlockChoice=Vector  SimViewingDevice=off
      link override Value: Value=AC.Aerodynamics.Side.CYdr
      link override Vector: Vector=AC.Aerodynamics.Roll.Clr
      settings: AttributesFormatString=%<BlockChoice>  TemplateBlock=aerosimlib/FlightGear-Compatible/Aerodynamics/Coefficient  MemberBlocks=Table,Value,Vector  Permissions=ReadWrite  RTWFcnNameOpts=Auto  RTWFileNameOpts=Auto
  Clr*r : Product  Inputs=2  Multiplication=Element-wise(.*)  SaturateOnIntegerOverflow=on
  Demux : Demux  Outputs=4  BusSelectionMode=off
  Demux1 : Demux  Outputs=3  BusSelectionMode=off
  Demux3 : Demux  Outputs=3  BusSelectionMode=off
  Sum : Sum  Inputs=++  SaturateOnIntegerOverflow=on
  Sum1 : Sum  Inputs=++++  SaturateOnIntegerOverflow=on
  Terminator2 : Terminator
  Terminator3 : Terminator
  Terminator4 : Terminator
  Wing span : Constant  Value=AC.Metrics.WingSpan
  Cl : Outport  Port=1
  wires:
  Demux3/3 -> Clr*r/2
  Demux3/1 -> Clp*p/2
  Clp*p/1 -> Sum/1
  Clr*r/1 -> Sum/2
  Clr/1(Coeff) -> Clr*r/1
  Clp/1(Coeff) -> Clp*p/1
  Sum1/1 -> Cl/1
  AngularRates/1 -> Demux3/1
  Control/1 -> Demux/1
  WindAxesVel/1 -> Demux1/1
  Wing span/1 -> Cl*b/(2V)/2
  2/1 -> Cl*b/(2V)/3
  Sum/1 -> Cl*b/(2V)/1
  Demux1/1 -> 2/1
  Demux1/2 -> Cl beta/1(RowParam)
  Demux/3 -> Cl aileron/1(RowParam)
  Demux/4 -> Cl rudder/1(RowParam)
  Demux3/2 -> Terminator4/1
  Demux1/3 -> Clr/1(RowParam), Clp/1(RowParam), Cl beta/2(ColParam)
  Demux/1 -> Terminator2/1
  Demux/2 -> Terminator3/1
  Cl beta/1(Coeff) -> Sum1/1
  Cl aileron/1(Coeff) -> Sum1/2
  Cl rudder/1(Coeff) -> Sum1/3
  Cl*b/(2V)/1 -> Sum1/4

== system tp333079/FlightGear-Compatible/Complete Aircraft/CESSNA-182/Aerodynamics/Side ==
  Control : Inport  Port=1  PortDimensions=[4 1]  SampleTime=-1  DataType=auto
      settings: SignalType=auto
  WindAxesVel : Inport  Port=2  PortDimensions=[3 1]  SampleTime=-1  DataType=auto
      settings: SignalType=auto
  AngularRates : Inport  Port=3  PortDimensions=[3 1]  SampleTime=-1  DataType=auto
      settings: SignalType=auto
  2 : Gain  Gain=2  Multiplication=Element-wise(K.*u)  SaturateOnIntegerOverflow=on
  CY aileron : Subsystem  BlockChoice=Value  SimViewingDevice=off
      link override Value: Value=AC.Aerodynamics.Side.CYDa
      settings: AttributesFormatString=%<BlockChoice>  TemplateBlock=aerosimlib/FlightGear-Compatible/Aerodynamics/Coefficient  MemberBlocks=Table,Value,Vector  Permissions=ReadWrite  RTWFcnNameOpts=Auto  RTWFileNameOpts=Auto
  CY beta : Subsystem  BlockChoice=Vector  SimViewingDevice=off
      link override Value: Value=AC.Aerodynamics.Lift.Basic.kCLge
      link override Vector: Vector=AC.Aerodynamics.Side.CYb
      settings: AttributesFormatString=%<BlockChoice>  TemplateBlock=aerosimlib/FlightGear-Compatible/Aerodynamics/Coefficient  MemberBlocks=Table,Value,Vector  Permissions=ReadWrite  RTWFcnNameOpts=Auto  RTWFileNameOpts=Auto
  CY rudder : Subsystem  BlockChoice=Value  SimViewingDevice=off
      link override Value: Value=AC.Aerodynamics.Side.CYDr
      settings: AttributesFormatString=%<BlockChoice>  TemplateBlock=aerosimlib/FlightGear-Compatible/Aerodynamics/Coefficient  MemberBlocks=Table,Value,Vector  Permissions=ReadWrite  RTWFcnNameOpts=Auto  RTWFileNameOpts=Auto
  CY*b/(2V) : Product  Inputs=**/  Multiplication=Element-wise(.*)  SaturateOnIntegerOverflow=on
  CYb*b : Product  Inputs=2  Multiplication=Element-wise(.*)  SaturateOnIntegerOverflow=on
  CYp : Subsystem  BlockChoice=Vector  SimViewingDevice=off
      link override Value: Value=AC.Aerodynamics.Side.CYp
      link override Vector: Vector=AC.Aerodynamics.Side.CYp
      settings: AttributesFormatString=%<BlockChoice>  TemplateBlock=aerosimlib/FlightGear-Compatible/Aerodynamics/Coefficient  MemberBlocks=Table,Value,Vector  Permissions=ReadWrite  RTWFcnNameOpts=Auto  RTWFileNameOpts=Auto
  CYp*p : Product  Inputs=2  Multiplication=Element-wise(.*)  SaturateOnIntegerOverflow=on
  CYr : Subsystem  BlockChoice=Vector  SimViewingDevice=off
      link override Value: Value=AC.Aerodynamics.Side.CYr
      link override Vector: Vector=AC.Aerodynamics.Side.CYr
      settings: AttributesFormatString=%<BlockChoice>  TemplateBlock=aerosimlib/FlightGear-Compatible/Aerodynamics/Coefficient  MemberBlocks=Table,Value,Vector  Permissions=ReadWrite  RTWFcnNameOpts=Auto  RTWFileNameOpts=Auto
  CYr*r : Product  Inputs=2  Multiplication=Element-wise(.*)  SaturateOnIntegerOverflow=on
  Demux : Demux  Outputs=4  BusSelectionMode=off
  Demux1 : Demux  Outputs=3  BusSelectionMode=off
  Demux3 : Demux  Outputs=3  BusSelectionMode=off
  Sum : Sum  Inputs=++  SaturateOnIntegerOverflow=on
  Sum1 : Sum  Inputs=++++  SaturateOnIntegerOverflow=on
  Terminator2 : Terminator
  Terminator3 : Terminator
  Terminator4 : Terminator
  Wing span : Constant  Value=AC.Metrics.WingSpan
  CY : Outport  Port=1
  wires:
  Demux3/3 -> CYr*r/2
  Demux3/1 -> CYp*p/2
  CYr*r/1 -> Sum/2
  CYr/1(Coeff) -> CYr*r/1
  CYp*p/1 -> Sum/1
  CYp/1(Coeff) -> CYp*p/1
  Demux1/2 -> CYb*b/2
  CYb*b/1 -> Sum1/1
  CY beta/1(Coeff) -> CYb*b/1
  CY*b/(2V)/1 -> Sum1/4
  CY rudder/1(Coeff) -> Sum1/3
  CY aileron/1(Coeff) -> Sum1/2
  Demux/2 -> Terminator3/1
  Demux/1 -> Terminator2/1
  Demux1/3 -> CYr/1(RowParam), CYp/1(RowParam), CY beta/1(RowParam)
  Demux3/2 -> Terminator4/1
  Demux/4 -> CY rudder/1(RowParam)
  Demux/3 -> CY aileron/1(RowParam)
  Demux1/1 -> 2/1
  Sum/1 -> CY*b/(2V)/1
  2/1 -> CY*b/(2V)/3
  Wing span/1 -> CY*b/(2V)/2
  WindAxesVel/1 -> Demux1/1
  Control/1 -> Demux/1
  AngularRates/1 -> Demux3/1
  Sum1/1 -> CY/1
